simulink model "Lab2_4"  (R2022b)
settings: Solver=VariableStepAuto  StartTime=0.0  StopTime=6  RelTol=1e-3
undefined symbols (not defined in the file): Bs, Ks, Kus, Ms, Mus
libraries: slpidlib x1
settings Model: Creator=Niku  LastModifiedBy=Niku
settings ModelReferenceCC: EnableRefExpFcnMdlSchedulingChecks=on

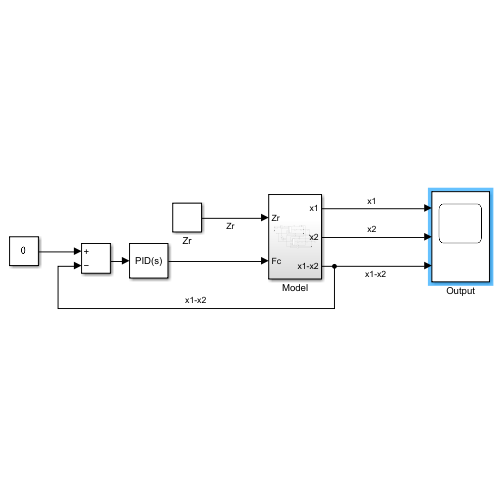
[thumbnail: Simulink's stored preview of the top-level diagram]
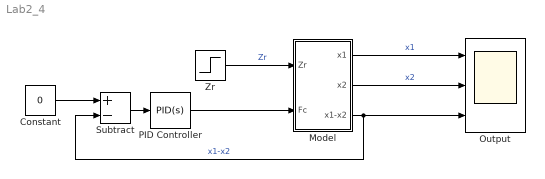
== system Lab2_4 ==
  Constant : Constant  Value=0
  Model : Subsystem
  Output : Scope  NumInputPorts=3
  PID Controller : slpidlib/PID Controller  Controller=PID  Form=Parallel  TimeDomain=Continuous-time  UseExternalTs=off  SampleTime=-1  IntegratorMethod=Forward Euler  FilterMethod=Forward Euler  ControllerParametersSource=internal  P=-2604342.42333957  I=-72208219.3953643  UseKiTs=off  D=-23206.9803615599  N=12371.0397061165  UseFilter=on  TunerSelectOption=Transfer Function Based (PID Tuner App)  InitialConditionSource=internal  InitialConditionForIntegrator=0  InitialConditionForFilter=0  DifferentiatorICPrevScaledInput=0  ExternalReset=none  TrackingMode=off  Kt=1  LimitOutput=off  SatLimitsSource=internal  UpperSaturationLimit=inf  LowerSaturationLimit=-inf  LinearizeAsGain=on  AntiWindupMode=none  Kb=1  LimitIntegrator=off  UpperIntegratorSaturationLimit=inf  LowerIntegratorSaturationLimit=-inf  POutMin=[]  POutMax=[]  IOutMin=[]  IOutMax=[]  DOutMin=[]  DOutMax=[]  NOutMin=[]  NOutMax=[]  SumOutMin=[]  SumOutMax=[]  SaturationOutMin=[]  SaturationOutMax=[]  PParamMin=[]  PParamMax=[]  IParamMin=[]  IParamMax=[]  DParamMin=[]  DParamMax=[]  NParamMin=[]  NParamMax=[]  KbParamMin=[]  KbParamMax=[]  KtParamMin=[]  KtParamMax=[]  KbOutMin=[]  KbOutMax=[]  KtOutMin=[]  KtOutMax=[]  IntegratorOutMin=[]  IntegratorOutMax=[]  FilterOutMin=[]  FilterOutMax=[]  SumI1OutMin=[]  SumI1OutMax=[]  SumI2OutMin=[]  SumI2OutMax=[]  SumI3OutMin=[]  SumI3OutMax=[]  SumI4OutMin=[]  SumI4OutMax=[]  SumDOutMin=[]  SumDOutMax=[]  DifferentiatorOutMin=[]  DifferentiatorOutMax=[]  FilterDiffOutCoefMin=[]  FilterDiffOutCoefMax=[]  ReciprocalOutMin=[]  ReciprocalOutMax=[]  SumDenOutMin=[]  SumDenOutMax=[]  SumNumOutMin=[]  SumNumOutMax=[]  DivideOutMin=[]  DivideOutMax=[]  UdiffTsProdOutMin=[]  UdiffTsProdOutMax=[]  NTsProdOutMin=[]  NTsProdOutMax=[]  UintegralTsProdOutMin=[]  UintegralTsProdOutMax=[]  UngainTsProdOutMin=[]  UngainTsProdOutMax=[]  ClampingZeroOutDataTypeStr=Inherit: Inherit via back propagation  ClampingZeroOutMin=[]  ClampingZeroOutMax=[]  FilterDenConstantOutDataTypeStr=Inherit: Inherit via back propagation  FilterDenConstantOutMin=[]  FilterDenConstantOutMax=[]  PCopyOutDataTypeStr=Inherit: Inherit via back propagation  PCopyOutMin=[]  PCopyOutMax=[]  NCopyOutDataTypeStr=Inherit: Inherit via back propagation  NCopyOutMin=[]  NCopyOutMax=[]  IntegratorContinuousStateAttributes=''  IntegratorStateMustResolveToSignalObject=off  IntegratorRTWStateStorageClass=Auto  FilterContinuousStateAttributes=''  FilterStateMustResolveToSignalObject=off  FilterRTWStateStorageClass=Auto  ParallelPVariant=InternalParameters  IdealPVariant=Disabled  IVariant=InternalParameters  DVariant=InternalParameters  IntegratorVariant=Continuous  SatVariant=Disabled  AWVariant=Passthrough  PCopyVariant=Disabled  TRVariant=Disabled  FdbkBlocksVariant=Forward  IdealPFdbkVariant=Disabled  SatFdbkVariant=Disabled  DerivativeFilterVariant=ContFilter  NVariant=InternalParameters  NCopyVariant=Disabled  FilterICVariant=InternalICsFilter  IntegratorICVariant=InternalICs  ExternalResetVariant=Disabled  TRSumVariant=Passthrough  SumFdbkVariant=Disabled  SumVariant=Sum_PID  TsampFilterVariant=InternalTs  TsampNgainVariant=Passthrough  TsampIntegralVariant=Passthrough  ExternalSaturationOutDataTypeStr=Inherit: Same as second input
  Subtract : Sum  Inputs=+-
  Zr : Step  After=0.1  SampleTime=0
  wires:
  PID Controller/1 -> Model/2(Fc)
  Zr/1 -> Model/1(Zr)  "Zr"
  Model/1(x1) -> Output/1  "x1"
  Model/2(x2) -> Output/2  "x2"
  Model/3(x1-x2) -> Output/3, Subtract/2  "x1-x2"
  Subtract/1 -> PID Controller/1
  Constant/1 -> Subtract/1

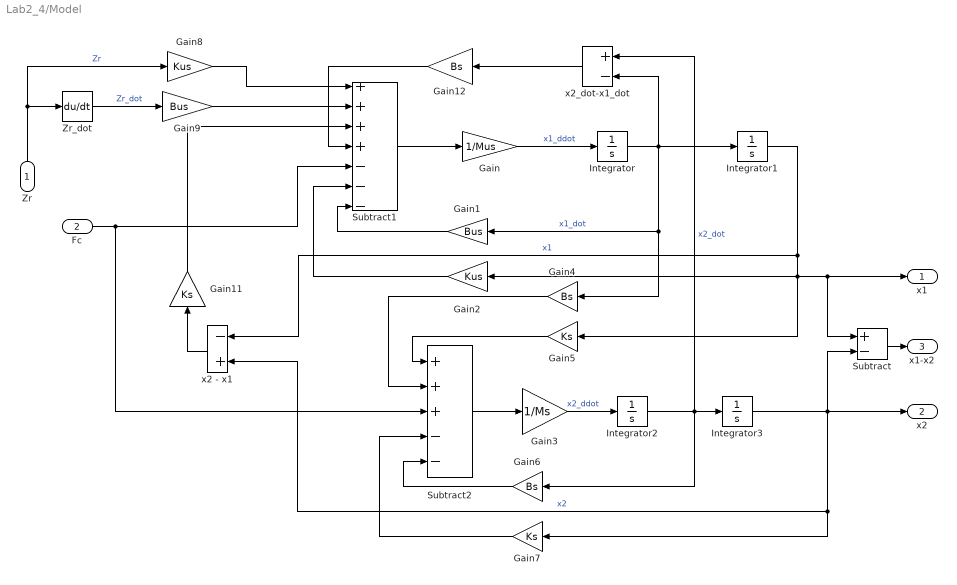
== system Lab2_4/Model ==
  Zr : Inport
  Fc : Inport  Port=2
  Gain : Gain  Gain=1/Mus
  Gain1 : Gain  Gain=Bus
  Gain11 : Gain  Gain=Ks
  Gain12 : Gain  Gain=Bs
  Gain2 : Gain  Gain=Kus
  Gain3 : Gain  Gain=1/Ms
  Gain4 : Gain  Gain=Bs
  Gain5 : Gain  Gain=Ks
  Gain6 : Gain  Gain=Bs
  Gain7 : Gain  Gain=Ks
  Gain8 : Gain  Gain=Kus
  Gain9 : Gain  Gain=Bus
  Integrator{,1..3} (4 alike) : Integrator
  Subtract : Sum  Inputs=+-
  Subtract1 : Sum  Inputs=++++---
  Subtract2 : Sum  Inputs=+++--
  Zr_dot : Derivative  CoefficientInTFapproximation=0
  x2 - x1 : Sum  Inputs=-+
  x2_dot-x1_dot : Sum  Inputs=+-
  x1 : Outport
  x2 : Outport  Port=2
  x1-x2 : Outport  Port=3
  wires:
  Gain5/1 -> Subtract2/1
  Gain11/1 -> Subtract1/3
  Gain8/1 -> Subtract1/1
  Gain9/1 -> Subtract1/2
  Integrator1/1 -> x2 - x1/1, Gain5/1, x1/1, Subtract/1, Gain2/1  "x1"
  Gain7/1 -> Subtract2/4
  Zr_dot/1 -> Gain9/1  "Zr_dot"
  Gain4/1 -> Subtract2/2
  Integrator2/1 -> Gain6/1, x2_dot-x1_dot/1, Integrator3/1  "x2_dot"
  Gain3/1 -> Integrator2/1  "x2_ddot"
  Gain/1 -> Integrator/1  "x1_ddot"
  Gain6/1 -> Subtract2/5
  Subtract2/1 -> Gain3/1
  Integrator/1 -> Gain4/1, Gain1/1, x2_dot-x1_dot/2, Integrator1/1  "x1_dot"
  Integrator3/1 -> x2/1, Subtract/2, x2 - x1/2, Gain7/1  "x2"
  Gain12/1 -> Subtract1/4
  Zr/1 -> Gain8/1, Zr_dot/1  "Zr"
  x2_dot-x1_dot/1 -> Gain12/1
  Subtract1/1 -> Gain/1
  Gain1/1 -> Subtract1/7
  Gain2/1 -> Subtract1/6
  x2 - x1/1 -> Gain11/1
  Fc/1 -> Subtract1/5, Subtract2/3
  Subtract/1 -> x1-x2/1
